simulink model "dinamica_quad"  (Simulink 7.6)
settings: Solver=ode45  StartTime=0.0  StopTime=10.0  MaxStep=0.1  RelTol=1e-3
values from neighbouring files (symbols this model uses):
  g = evalin('base','g')    [f.m]
  Ixx = evalin('base','Ixx')    [f.m]
  Iyy = evalin('base','Iyy')    [f.m]
  Izz = evalin('base','Izz')    [f.m]
  Izzm = evalin('base','Izzm')    [f.m]
  L = evalin('base','L')    [f.m]
  M = evalin('base','M')    [f.m]
  phi0 = evalin('base','phi0')    [determinar_vel.m]
  psi0 = evalin('base','psi0')    [determinar_vel.m]
  theta0 = evalin('base','theta0')    [determinar_vel.m]
undefined symbols (not defined in the file or in its folder): vq10, vq20, vq30, wq10, wq20, wq30, x0, y0, z0
settings Model: Creator=pater  LastModifiedBy=pater

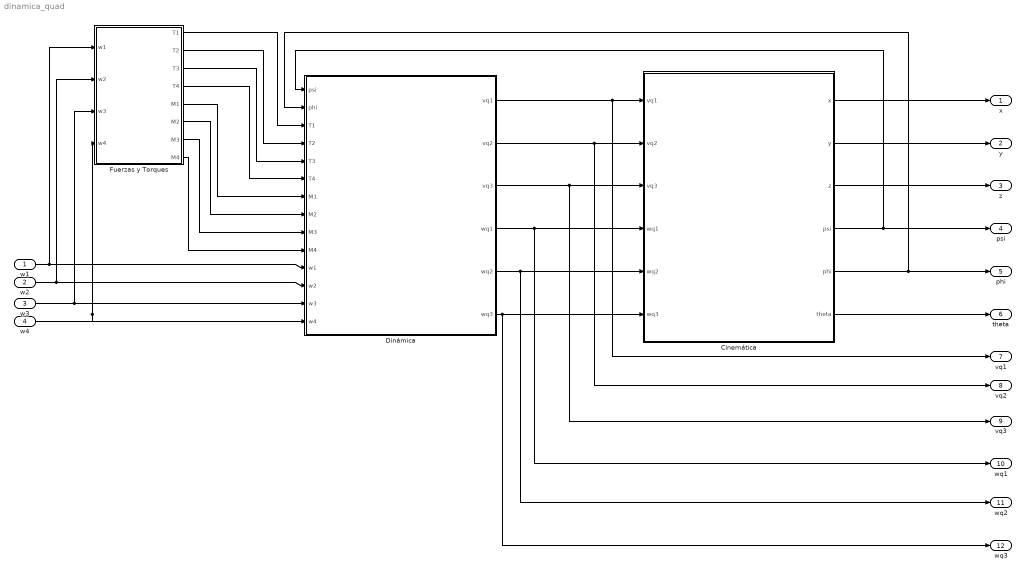
== system dinamica_quad ==
  w1 : Inport
  w2 : Inport  Port=2
  w3 : Inport  Port=3
  w4 : Inport  Port=4
  Cinemática : Subsystem
  Dinámica : Subsystem
  Fuerzas y Torques : Subsystem
  x : Outport
  y : Outport  Port=2
  z : Outport  Port=3
  psi : Outport  Port=4
  phi : Outport  Port=5
  theta : Outport  Port=6
  vq1 : Outport  Port=7
  vq2 : Outport  Port=8
  vq3 : Outport  Port=9
  wq1 : Outport  Port=10
  wq2 : Outport  Port=11
  wq3 : Outport  Port=12
  wires:
  Cinemática/1(x) -> x/1
  Cinemática/2(y) -> y/1
  Cinemática/3(z) -> z/1
  Cinemática/4(psi) -> psi/1, Dinámica/1(psi)
  Cinemática/5(phi) -> phi/1, Dinámica/2(phi)
  Cinemática/6(theta) -> theta/1
  w2/1 -> Fuerzas y Torques/2(w2), Dinámica/12(w2)
  w3/1 -> Fuerzas y Torques/3(w3), Dinámica/13(w3)
  w4/1 -> Fuerzas y Torques/4(w4), Dinámica/14(w4)
  Dinámica/6(wq3) -> wq3/1, Cinemática/6(wq3)
  Fuerzas y Torques/1(T1) -> Dinámica/3(T1)
  Fuerzas y Torques/2(T2) -> Dinámica/4(T2)
  Fuerzas y Torques/3(T3) -> Dinámica/5(T3)
  Fuerzas y Torques/4(T4) -> Dinámica/6(T4)
  Fuerzas y Torques/5(M1) -> Dinámica/7(M1)
  Fuerzas y Torques/6(M2) -> Dinámica/8(M2)
  Fuerzas y Torques/7(M3) -> Dinámica/9(M3)
  Fuerzas y Torques/8(M4) -> Dinámica/10(M4)
  w1/1 -> Fuerzas y Torques/1(w1), Dinámica/11(w1)
  Dinámica/1(vq1) -> Cinemática/1(vq1), vq1/1
  Dinámica/2(vq2) -> Cinemática/2(vq2), vq2/1
  Dinámica/3(vq3) -> Cinemática/3(vq3), vq3/1
  Dinámica/4(wq1) -> Cinemática/4(wq1), wq1/1
  Dinámica/5(wq2) -> Cinemática/5(wq2), wq2/1

== system dinamica_quad/Cinemática ==
  vq1 : Inport
  vq2 : Inport  Port=2
  vq3 : Inport  Port=3
  wq1 : Inport  Port=4
  wq2 : Inport  Port=5
  wq3 : Inport  Port=6
  Posiciones : Subsystem
  Ángulos De Euler : Subsystem
  x : Outport
  y : Outport  Port=2
  z : Outport  Port=3
  psi : Outport  Port=4
  phi : Outport  Port=5
  theta : Outport  Port=6
  wires:
  Posiciones/1(x) -> x/1
  Posiciones/2(y) -> y/1
  Posiciones/3(z) -> z/1
  Ángulos De Euler/1(psi) -> psi/1, Posiciones/3(psi)
  Ángulos De Euler/2(phi) -> phi/1, Posiciones/2(phi)
  Ángulos De Euler/3(theta) -> theta/1, Posiciones/1(theta)
  vq1/1 -> Posiciones/4(vq1)
  vq2/1 -> Posiciones/5(vq2)
  vq3/1 -> Posiciones/6(vq3)
  wq1/1 -> Ángulos De Euler/1(wq1)
  wq2/1 -> Ángulos De Euler/2(wq2)
  wq3/1 -> Ángulos De Euler/3(wq3)

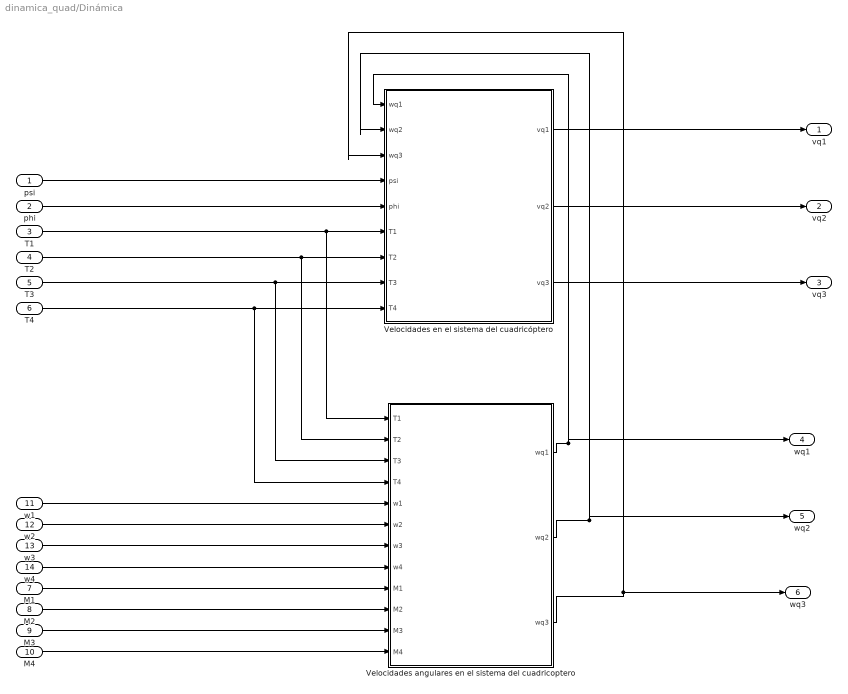
== system dinamica_quad/Dinámica ==
  psi : Inport
  phi : Inport  Port=2
  T1 : Inport  Port=3
  T2 : Inport  Port=4
  T3 : Inport  Port=5
  T4 : Inport  Port=6
  M1 : Inport  Port=7
  M2 : Inport  Port=8
  M3 : Inport  Port=9
  M4 : Inport  Port=10
  w1 : Inport  Port=11
  w2 : Inport  Port=12
  w3 : Inport  Port=13
  w4 : Inport  Port=14
  Velocidades angulares en el sistema del cuadricoptero : Subsystem
  Velocidades en el sistema del cuadricóptero : Subsystem
  vq1 : Outport
  vq2 : Outport  Port=2
  vq3 : Outport  Port=3
  wq1 : Outport  Port=4
  wq2 : Outport  Port=5
  wq3 : Outport  Port=6
  wires:
  T1/1 -> Velocidades en el sistema del cuadricóptero/6(T1), Velocidades angulares en el sistema del cuadricoptero/1(T1)
  T2/1 -> Velocidades en el sistema del cuadricóptero/7(T2), Velocidades angulares en el sistema del cuadricoptero/2(T2)
  T3/1 -> Velocidades en el sistema del cuadricóptero/8(T3), Velocidades angulares en el sistema del cuadricoptero/3(T3)
  T4/1 -> Velocidades en el sistema del cuadricóptero/9(T4), Velocidades angulares en el sistema del cuadricoptero/4(T4)
  Velocidades angulares en el sistema del cuadricoptero/1(wq1) -> wq1/1, Velocidades en el sistema del cuadricóptero/1(wq1)
  Velocidades angulares en el sistema del cuadricoptero/2(wq2) -> wq2/1, Velocidades en el sistema del cuadricóptero/2(wq2)
  Velocidades angulares en el sistema del cuadricoptero/3(wq3) -> Velocidades en el sistema del cuadricóptero/3(wq3), wq3/1
  phi/1 -> Velocidades en el sistema del cuadricóptero/5(phi)
  psi/1 -> Velocidades en el sistema del cuadricóptero/4(psi)
  Velocidades en el sistema del cuadricóptero/3(vq3) -> vq3/1
  Velocidades en el sistema del cuadricóptero/2(vq2) -> vq2/1
  Velocidades en el sistema del cuadricóptero/1(vq1) -> vq1/1
  M2/1 -> Velocidades angulares en el sistema del cuadricoptero/10(M2)
  M3/1 -> Velocidades angulares en el sistema del cuadricoptero/11(M3)
  M4/1 -> Velocidades angulares en el sistema del cuadricoptero/12(M4)
  M1/1 -> Velocidades angulares en el sistema del cuadricoptero/9(M1)
  w1/1 -> Velocidades angulares en el sistema del cuadricoptero/5(w1)
  w2/1 -> Velocidades angulares en el sistema del cuadricoptero/6(w2)
  w3/1 -> Velocidades angulares en el sistema del cuadricoptero/7(w3)
  w4/1 -> Velocidades angulares en el sistema del cuadricoptero/8(w4)

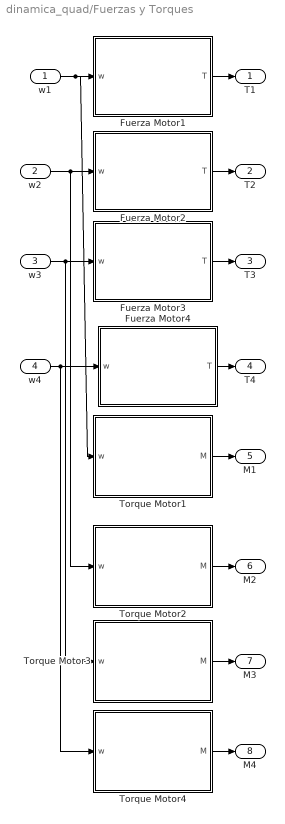
== system dinamica_quad/Fuerzas y Torques ==
  w1 : Inport
  w2 : Inport  Port=2
  w3 : Inport  Port=3
  w4 : Inport  Port=4
  Fuerza Motor1 : Subsystem
  Fuerza Motor2 : Subsystem
  Fuerza Motor3 : Subsystem
  Fuerza Motor4 : Subsystem
  Torque Motor1 : Subsystem
  Torque Motor2 : Subsystem
  Torque Motor3 : Subsystem
  Torque Motor4 : Subsystem
  T1 : Outport
  T2 : Outport  Port=2
  T3 : Outport  Port=3
  T4 : Outport  Port=4
  M1 : Outport  Port=5
  M2 : Outport  Port=6
  M3 : Outport  Port=7
  M4 : Outport  Port=8
  wires:
  w1/1 -> Fuerza Motor1/1(w), Torque Motor1/1(w)
  w2/1 -> Fuerza Motor2/1(w), Torque Motor2/1(w)
  w3/1 -> Fuerza Motor3/1(w), Torque Motor3/1(w)
  w4/1 -> Fuerza Motor4/1(w), Torque Motor4/1(w)
  Fuerza Motor1/1(T) -> T1/1
  Fuerza Motor2/1(T) -> T2/1
  Fuerza Motor3/1(T) -> T3/1
  Fuerza Motor4/1(T) -> T4/1
  Torque Motor1/1(M) -> M1/1
  Torque Motor2/1(M) -> M2/1
  Torque Motor3/1(M) -> M3/1
  Torque Motor4/1(M) -> M4/1

== system dinamica_quad/Cinemática/Posiciones ==
  theta : Inport
  phi : Inport  Port=2
  psi : Inport  Port=3
  vq1 : Inport  Port=4
  vq2 : Inport  Port=5
  vq3 : Inport  Port=6
  Subsystem3 : Subsystem
  Subsystem4 : Subsystem
  Subsystem5 : Subsystem
  x : Outport
  y : Outport  Port=2
  z : Outport  Port=3
  wires:
  Subsystem3/1(x) -> x/1
  Subsystem4/1(y) -> y/1
  Subsystem5/1(z) -> z/1
  vq3/1 -> Subsystem5/5(vq3), Subsystem4/6(vq3), Subsystem3/6(vq3)
  theta/1 -> Subsystem3/1(theta), Subsystem4/1(theta)
  phi/1 -> Subsystem3/2(phi), Subsystem4/2(phi), Subsystem5/1(phi)
  psi/1 -> Subsystem3/3(psi), Subsystem4/3(psi), Subsystem5/2(psi)
  vq2/1 -> Subsystem5/4(vq2), Subsystem4/5(vq2), Subsystem3/5(vq2)
  vq1/1 -> Subsystem5/3(vq1), Subsystem4/4(vq1), Subsystem3/4(vq1)

== system dinamica_quad/Cinemática/Ángulos De Euler ==
  wq1 : Inport
  wq2 : Inport  Port=2
  wq3 : Inport  Port=3
  Subsystem : Subsystem
  Subsystem1 : Subsystem
  Subsystem2 : Subsystem
  psi : Outport
  phi : Outport  Port=2
  theta : Outport  Port=3
  wires:
  Subsystem1/1(psi) -> psi/1, Subsystem/1(psi), Subsystem2/1(psi)
  Subsystem2/1(phi) -> phi/1, Subsystem/2(phi), Subsystem1/1(phi)
  Subsystem/1(theta) -> theta/1
  wq3/1 -> Subsystem/4(wq3), Subsystem2/3(wq3), Subsystem1/2(wq3)
  wq1/1 -> Subsystem1/4(wq1)
  wq2/1 -> Subsystem2/2(wq2), Subsystem1/3(wq2), Subsystem/3(wq2)

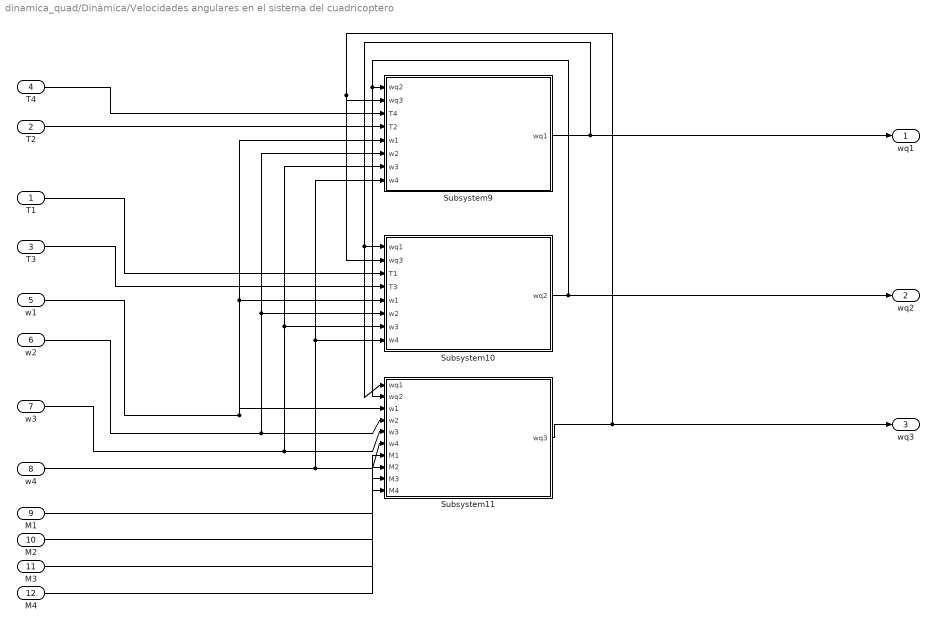
== system dinamica_quad/Dinámica/Velocidades angulares en el sistema del cuadricoptero ==
  T1 : Inport
  T2 : Inport  Port=2
  T3 : Inport  Port=3
  T4 : Inport  Port=4
  w1 : Inport  Port=5
  w2 : Inport  Port=6
  w3 : Inport  Port=7
  w4 : Inport  Port=8
  M1 : Inport  Port=9
  M2 : Inport  Port=10
  M3 : Inport  Port=11
  M4 : Inport  Port=12
  Subsystem10 : Subsystem
  Subsystem11 : Subsystem
  Subsystem9 : Subsystem
  wq1 : Outport
  wq2 : Outport  Port=2
  wq3 : Outport  Port=3
  wires:
  Subsystem9/1(wq1) -> wq1/1, Subsystem11/1(wq1), Subsystem10/1(wq1)
  Subsystem10/1(wq2) -> wq2/1, Subsystem11/2(wq2), Subsystem9/1(wq2)
  Subsystem11/1(wq3) -> wq3/1, Subsystem10/2(wq3), Subsystem9/2(wq3)
  w4/1 -> Subsystem11/6(w4), Subsystem10/8(w4), Subsystem9/8(w4)
  w3/1 -> Subsystem11/5(w3), Subsystem10/7(w3), Subsystem9/7(w3)
  w2/1 -> Subsystem11/4(w2), Subsystem10/6(w2), Subsystem9/6(w2)
  w1/1 -> Subsystem11/3(w1), Subsystem10/5(w1), Subsystem9/5(w1)
  T3/1 -> Subsystem10/4(T3)
  T1/1 -> Subsystem10/3(T1)
  T2/1 -> Subsystem9/4(T2)
  T4/1 -> Subsystem9/3(T4)
  M1/1 -> Subsystem11/7(M1)
  M2/1 -> Subsystem11/8(M2)
  M3/1 -> Subsystem11/9(M3)
  M4/1 -> Subsystem11/10(M4)

== system dinamica_quad/Dinámica/Velocidades en el sistema del cuadricóptero ==
  wq1 : Inport
  wq2 : Inport  Port=2
  wq3 : Inport  Port=3
  psi : Inport  Port=4
  phi : Inport  Port=5
  T1 : Inport  Port=6
  T2 : Inport  Port=7
  T3 : Inport  Port=8
  T4 : Inport  Port=9
  Subsystem6 : Subsystem
  Subsystem7 : Subsystem
  Subsystem8 : Subsystem
  vq1 : Outport
  vq2 : Outport  Port=2
  vq3 : Outport  Port=3
  wires:
  Subsystem6/1(vq1) -> vq1/1, Subsystem8/5(vq1), Subsystem7/7(vq1), Subsystem7/8(vq2)
  Subsystem8/1(vq2) -> Subsystem6/4(vq2), vq2/1
  Subsystem7/1(vq3) -> vq3/1, Subsystem6/5(vq3), Subsystem8/4(vq3)
  wq1/1 -> Subsystem8/3(wq1), Subsystem7/1(wq1)
  wq3/1 -> Subsystem6/3(wq3), Subsystem8/2(wq3)
  psi/1 -> Subsystem8/6(psi), Subsystem7/10(psi)
  phi/1 -> Subsystem6/1(phi), Subsystem8/1(phi), Subsystem7/9(phi)
  wq2/1 -> Subsystem6/2(wq2), Subsystem7/2(wq2)
  T1/1 -> Subsystem7/3(T1)
  T2/1 -> Subsystem7/4(T2)
  T3/1 -> Subsystem7/5(T3)
  T4/1 -> Subsystem7/6(T4)

== system dinamica_quad/Fuerzas y Torques/Fuerza Motor1 ==
  w : Inport
  Add : Sum
  Gain : Gain  Gain=3.5296e-5
  Gain1 : Gain  Gain=-4.9293e-4
  Product : Product  RndMeth=Zero
  T : Outport
  wires:
  Add/1 -> T/1
  Gain1/1 -> Add/2
  Product/1 -> Gain/1
  Gain/1 -> Add/1
  w/1 -> Gain1/1, Product/2, Product/1

== system dinamica_quad/Fuerzas y Torques/Fuerza Motor2 ==
  w : Inport
  Add : Sum
  Gain : Gain  Gain=3.5296e-5
  Gain1 : Gain  Gain=-4.9293e-4
  Product : Product  RndMeth=Zero
  T : Outport
  wires:
  Add/1 -> T/1
  Gain1/1 -> Add/2
  Product/1 -> Gain/1
  Gain/1 -> Add/1
  w/1 -> Gain1/1, Product/2, Product/1

== system dinamica_quad/Fuerzas y Torques/Fuerza Motor3 ==
  w : Inport
  Add : Sum
  Gain : Gain  Gain=3.5296e-5
  Gain1 : Gain  Gain=-4.9293e-4
  Product : Product  RndMeth=Zero
  T : Outport
  wires:
  Add/1 -> T/1
  Gain1/1 -> Add/2
  Product/1 -> Gain/1
  Gain/1 -> Add/1
  w/1 -> Gain1/1, Product/2, Product/1

== system dinamica_quad/Fuerzas y Torques/Fuerza Motor4 ==
  w : Inport
  Add : Sum
  Gain : Gain  Gain=3.5296e-5
  Gain1 : Gain  Gain=-4.9293e-4
  Product : Product  RndMeth=Zero
  T : Outport
  wires:
  Add/1 -> T/1
  Gain1/1 -> Add/2
  Product/1 -> Gain/1
  Gain/1 -> Add/1
  w/1 -> Gain1/1, Product/2, Product/1

== system dinamica_quad/Fuerzas y Torques/Torque Motor1 ==
  w : Inport
  Add : Sum
  Gain : Gain  Gain=3.4734e-6
  Gain1 : Gain  Gain=-1.3205e-4
  Product : Product  RndMeth=Zero
  M : Outport
  wires:
  Add/1 -> M/1
  Gain1/1 -> Add/2
  Product/1 -> Gain/1
  Gain/1 -> Add/1
  w/1 -> Gain1/1, Product/2, Product/1

== system dinamica_quad/Fuerzas y Torques/Torque Motor2 ==
  w : Inport
  Add : Sum
  Gain : Gain  Gain=3.4734e-6
  Gain1 : Gain  Gain=-1.3205e-4
  Product : Product  RndMeth=Zero
  M : Outport
  wires:
  Add/1 -> M/1
  Gain1/1 -> Add/2
  Product/1 -> Gain/1
  Gain/1 -> Add/1
  w/1 -> Gain1/1, Product/2, Product/1

== system dinamica_quad/Fuerzas y Torques/Torque Motor3 ==
  w : Inport
  Add : Sum
  Gain : Gain  Gain=3.4734e-6
  Gain1 : Gain  Gain=-1.3205e-4
  Product : Product  RndMeth=Zero
  M : Outport
  wires:
  Add/1 -> M/1
  Gain1/1 -> Add/2
  Product/1 -> Gain/1
  Gain/1 -> Add/1
  w/1 -> Gain1/1, Product/2, Product/1

== system dinamica_quad/Fuerzas y Torques/Torque Motor4 ==
  w : Inport
  Add : Sum
  Gain : Gain  Gain=3.4734e-6
  Gain1 : Gain  Gain=-1.3205e-4
  Product : Product  RndMeth=Zero
  M : Outport
  wires:
  Add/1 -> M/1
  Gain1/1 -> Add/2
  Product/1 -> Gain/1
  Gain/1 -> Add/1
  w/1 -> Gain1/1, Product/2, Product/1

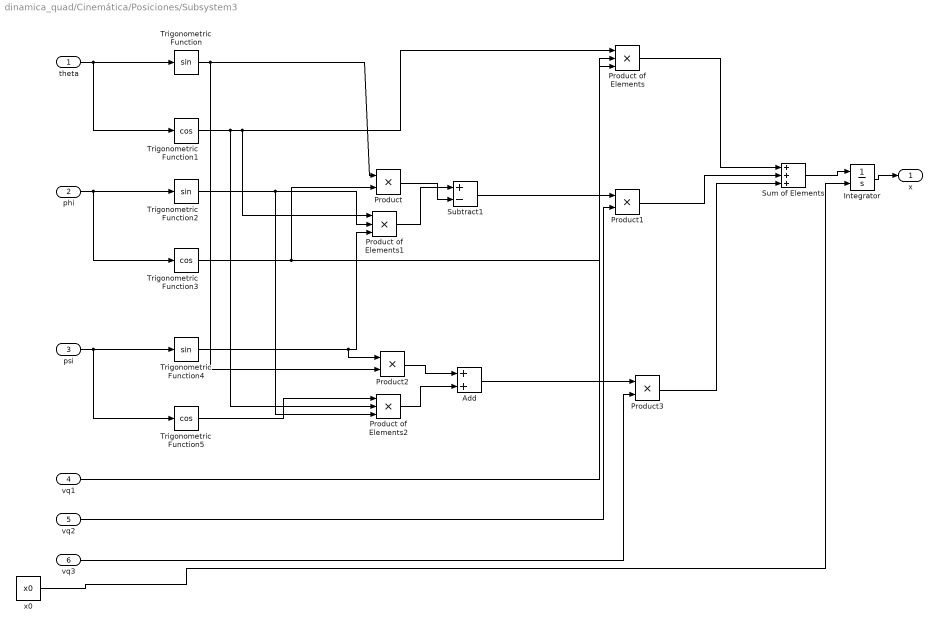
== system dinamica_quad/Cinemática/Posiciones/Subsystem3 ==
  theta : Inport
  phi : Inport  Port=2
  psi : Inport  Port=3
  vq1 : Inport  Port=4
  vq2 : Inport  Port=5
  vq3 : Inport  Port=6
  Add : Sum
  Integrator : Integrator  InitialConditionSource=external
  Product{,1..3} (4 alike) : Product  RndMeth=Zero
  Product of Elements : Product  Inputs=3
  Product of Elements1 : Product  Inputs=3
  Product of Elements2 : Product  Inputs=3
  Subtract1 : Sum  Inputs=+-
  Sum of Elements : Sum  Inputs=3
  Trigonometric Function : Trigonometry
  Trigonometric Function1 : Trigonometry  Operator=cos
  Trigonometric Function2 : Trigonometry
  Trigonometric Function3 : Trigonometry  Operator=cos
  Trigonometric Function4 : Trigonometry
  Trigonometric Function5 : Trigonometry  Operator=cos
  x0 : Constant  Value=x0
  x : Outport
  wires:
  theta/1 -> Trigonometric Function/1, Trigonometric Function1/1
  phi/1 -> Trigonometric Function2/1, Trigonometric Function3/1
  psi/1 -> Trigonometric Function4/1, Trigonometric Function5/1
  Trigonometric Function1/1 -> Product of Elements/1, Product of Elements1/1, Product of Elements2/2
  Trigonometric Function3/1 -> Product of Elements/2, Product/2
  vq1/1 -> Product of Elements/3
  Trigonometric Function/1 -> Product/1, Product2/2
  Trigonometric Function2/1 -> Product of Elements1/2, Product of Elements2/3
  Trigonometric Function4/1 -> Product of Elements1/3, Product2/1
  Subtract1/1 -> Product1/1
  vq2/1 -> Product1/2
  Product2/1 -> Add/1
  Product of Elements2/1 -> Add/2
  Trigonometric Function5/1 -> Product of Elements2/1
  Add/1 -> Product3/1
  vq3/1 -> Product3/2
  Product of Elements/1 -> Sum of Elements/1
  Product1/1 -> Sum of Elements/2
  Product3/1 -> Sum of Elements/3
  Sum of Elements/1 -> Integrator/1
  Integrator/1 -> x/1
  Product of Elements1/1 -> Subtract1/1
  Product/1 -> Subtract1/2
  x0/1 -> Integrator/2

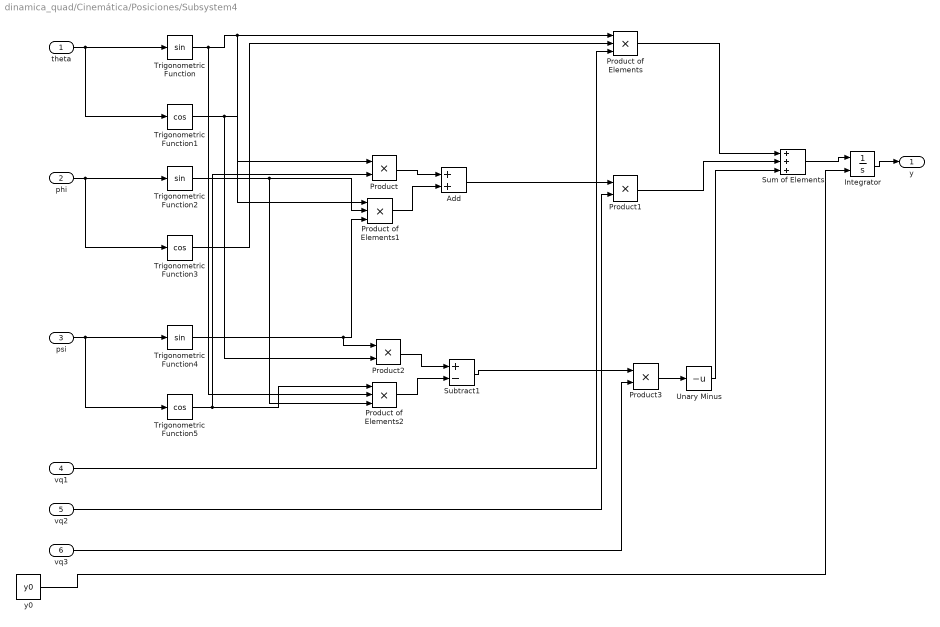
== system dinamica_quad/Cinemática/Posiciones/Subsystem4 ==
  theta : Inport
  phi : Inport  Port=2
  psi : Inport  Port=3
  vq1 : Inport  Port=4
  vq2 : Inport  Port=5
  vq3 : Inport  Port=6
  Add : Sum
  Integrator : Integrator  InitialConditionSource=external
  Product{,1..3} (4 alike) : Product  RndMeth=Zero
  Product of Elements : Product  Inputs=3
  Product of Elements1 : Product  Inputs=3
  Product of Elements2 : Product  Inputs=3
  Subtract1 : Sum  Inputs=+-
  Sum of Elements : Sum  Inputs=3
  Trigonometric Function : Trigonometry
  Trigonometric Function1 : Trigonometry  Operator=cos
  Trigonometric Function2 : Trigonometry
  Trigonometric Function3 : Trigonometry  Operator=cos
  Trigonometric Function4 : Trigonometry
  Trigonometric Function5 : Trigonometry  Operator=cos
  Unary Minus : UnaryMinus
  y0 : Constant  Value=y0
  y : Outport
  wires:
  theta/1 -> Trigonometric Function/1, Trigonometric Function1/1
  phi/1 -> Trigonometric Function2/1, Trigonometric Function3/1
  psi/1 -> Trigonometric Function4/1, Trigonometric Function5/1
  Trigonometric Function1/1 -> Product/1, Product2/2
  Trigonometric Function3/1 -> Product of Elements/2
  vq1/1 -> Product of Elements/3
  Trigonometric Function/1 -> Product of Elements/1, Product of Elements1/1, Product of Elements2/2
  Trigonometric Function2/1 -> Product of Elements1/2, Product of Elements2/3
  Trigonometric Function4/1 -> Product of Elements1/3, Product2/1
  Product/1 -> Add/1
  Product of Elements1/1 -> Add/2
  Add/1 -> Product1/1
  vq2/1 -> Product1/2
  Trigonometric Function5/1 -> Product of Elements2/1, Product/2
  Subtract1/1 -> Product3/1
  vq3/1 -> Product3/2
  Product of Elements/1 -> Sum of Elements/1
  Product1/1 -> Sum of Elements/2
  Product3/1 -> Unary Minus/1
  Sum of Elements/1 -> Integrator/1
  Integrator/1 -> y/1
  Unary Minus/1 -> Sum of Elements/3
  Product of Elements2/1 -> Subtract1/2
  Product2/1 -> Subtract1/1
  y0/1 -> Integrator/2

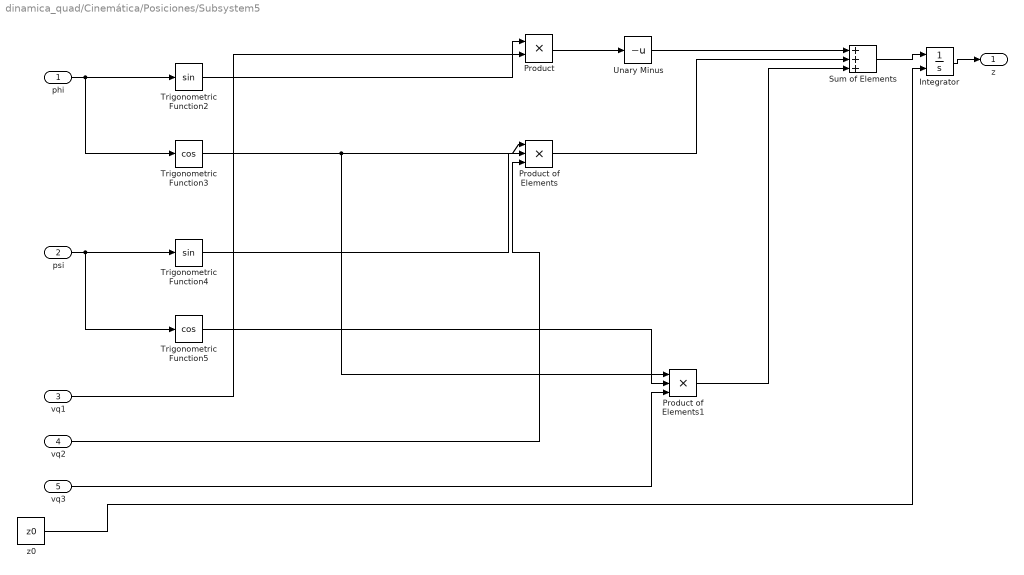
== system dinamica_quad/Cinemática/Posiciones/Subsystem5 ==
  phi : Inport
  psi : Inport  Port=2
  vq1 : Inport  Port=3
  vq2 : Inport  Port=4
  vq3 : Inport  Port=5
  Integrator : Integrator  InitialConditionSource=external
  Product : Product  RndMeth=Zero
  Product of Elements : Product  Inputs=3
  Product of Elements1 : Product  Inputs=3
  Sum of Elements : Sum  Inputs=3
  Trigonometric Function2 : Trigonometry
  Trigonometric Function3 : Trigonometry  Operator=cos
  Trigonometric Function4 : Trigonometry
  Trigonometric Function5 : Trigonometry  Operator=cos
  Unary Minus : UnaryMinus
  z0 : Constant  Value=z0
  z : Outport
  wires:
  phi/1 -> Trigonometric Function2/1, Trigonometric Function3/1
  psi/1 -> Trigonometric Function4/1, Trigonometric Function5/1
  Sum of Elements/1 -> Integrator/1
  Integrator/1 -> z/1
  Trigonometric Function2/1 -> Product/1
  vq1/1 -> Product/2
  Product/1 -> Unary Minus/1
  Trigonometric Function3/1 -> Product of Elements/1, Product of Elements1/1
  Trigonometric Function4/1 -> Product of Elements/2
  vq2/1 -> Product of Elements/3
  Trigonometric Function5/1 -> Product of Elements1/2
  vq3/1 -> Product of Elements1/3
  Product of Elements/1 -> Sum of Elements/2
  Product of Elements1/1 -> Sum of Elements/3
  Unary Minus/1 -> Sum of Elements/1
  z0/1 -> Integrator/2

== system dinamica_quad/Cinemática/Ángulos De Euler/Subsystem ==
  psi : Inport
  phi : Inport  Port=2
  wq2 : Inport  Port=3
  wq3 : Inport  Port=4
  Divide : Product  Inputs=*/
  Integrator : Integrator  InitialConditionSource=external
  Product : Product  RndMeth=Zero
  Product1 : Product  RndMeth=Zero
  Sum : Sum  Inputs=|++
  Trigonometric Function : Trigonometry  Operator=cos
  Trigonometric Function1 : Trigonometry
  Trigonometric Function2 : Trigonometry  Operator=cos
  theta0 : Constant  Value=theta0
  theta : Outport
  wires:
  wq3/1 -> Product/1
  wq2/1 -> Product1/1
  Product/1 -> Sum/1
  Product1/1 -> Sum/2
  Sum/1 -> Divide/1
  Trigonometric Function2/1 -> Divide/2
  Divide/1 -> Integrator/1
  Trigonometric Function/1 -> Product/2
  Trigonometric Function1/1 -> Product1/2
  phi/1 -> Trigonometric Function2/1
  Integrator/1 -> theta/1
  psi/1 -> Trigonometric Function/1, Trigonometric Function1/1
  theta0/1 -> Integrator/2

== system dinamica_quad/Cinemática/Ángulos De Euler/Subsystem1 ==
  phi : Inport
  wq3 : Inport  Port=2
  wq2 : Inport  Port=3
  wq1 : Inport  Port=4
  Add : Sum
  Integrator : Integrator  InitialConditionSource=external
  Product : Product  RndMeth=Zero
  Product1 : Product  RndMeth=Zero
  Product2 : Product  RndMeth=Zero
  Sum : Sum  Inputs=|++
  Trigonometric Function : Trigonometry
  Trigonometric Function2 : Trigonometry  Operator=tan
  Trigonometric Function3 : Trigonometry  Operator=cos
  psi0 : Constant  Value=psi0
  psi : Outport
  wires:
  Integrator/1 -> psi/1, Trigonometric Function3/1, Trigonometric Function/1
  Product/1 -> Sum/1
  phi/1 -> Trigonometric Function2/1
  Trigonometric Function2/1 -> Product/2
  wq3/1 -> Product1/2
  Trigonometric Function3/1 -> Product1/1
  Product1/1 -> Add/1
  Add/1 -> Product/1
  Trigonometric Function/1 -> Product2/1
  wq2/1 -> Product2/2
  Product2/1 -> Add/2
  wq1/1 -> Sum/2
  Sum/1 -> Integrator/1
  psi0/1 -> Integrator/2

== system dinamica_quad/Cinemática/Ángulos De Euler/Subsystem2 ==
  psi : Inport
  wq2 : Inport  Port=2
  wq3 : Inport  Port=3
  Integrator : Integrator  InitialConditionSource=external
  Product : Product  RndMeth=Zero
  Product1 : Product  RndMeth=Zero
  Subtract : Sum  Inputs=+-
  Trigonometric Function : Trigonometry  Operator=cos
  Trigonometric Function1 : Trigonometry
  phi0 : Constant  Value=phi0
  phi : Outport
  wires:
  Integrator/1 -> phi/1
  Subtract/1 -> Integrator/1
  Product/1 -> Subtract/1
  Product1/1 -> Subtract/2
  Trigonometric Function/1 -> Product/1
  psi/1 -> Trigonometric Function/1, Trigonometric Function1/1
  Trigonometric Function1/1 -> Product1/1
  wq2/1 -> Product/2
  wq3/1 -> Product1/2
  phi0/1 -> Integrator/2

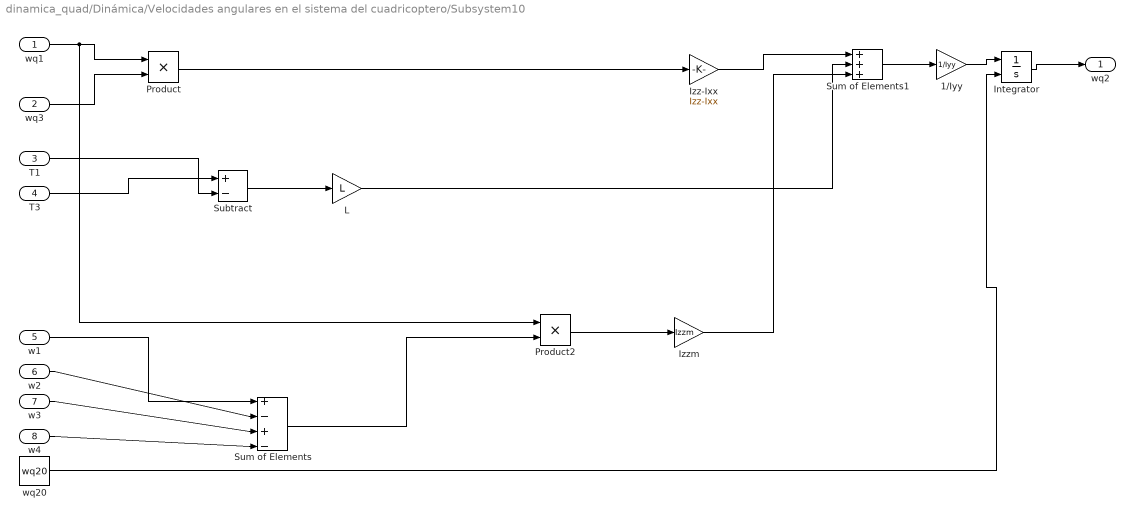
== system dinamica_quad/Dinámica/Velocidades angulares en el sistema del cuadricoptero/Subsystem10 ==
  wq1 : Inport
  wq3 : Inport  Port=2
  T1 : Inport  Port=3
  T3 : Inport  Port=4
  w1 : Inport  Port=5
  w2 : Inport  Port=6
  w3 : Inport  Port=7
  w4 : Inport  Port=8
  1/Iyy : Gain  Gain=1/Iyy
  Integrator : Integrator  InitialConditionSource=external
  Izz-Ixx : Gain  Gain=Izz-Ixx
  Izzm : Gain  Gain=Izzm
  L : Gain  Gain=L
  Product : Product  RndMeth=Zero
  Product2 : Product  RndMeth=Zero
  Subtract : Sum  Inputs=+-
  Sum of Elements : Sum  Inputs=+|-|+|-|
  Sum of Elements1 : Sum  Inputs=3
  wq20 : Constant  Value=wq20
  wq2 : Outport
  wires:
  wq1/1 -> Product/1, Product2/1
  wq3/1 -> Product/2
  Product/1 -> Izz-Ixx/1
  T3/1 -> Subtract/1
  T1/1 -> Subtract/2
  w1/1 -> Sum of Elements/1
  w2/1 -> Sum of Elements/2
  w3/1 -> Sum of Elements/3
  w4/1 -> Sum of Elements/4
  Sum of Elements/1 -> Product2/2
  Product2/1 -> Izzm/1
  Izzm/1 -> Sum of Elements1/3
  Sum of Elements1/1 -> 1/Iyy/1
  1/Iyy/1 -> Integrator/1
  Integrator/1 -> wq2/1
  Subtract/1 -> L/1
  Izz-Ixx/1 -> Sum of Elements1/1
  L/1 -> Sum of Elements1/2
  wq20/1 -> Integrator/2

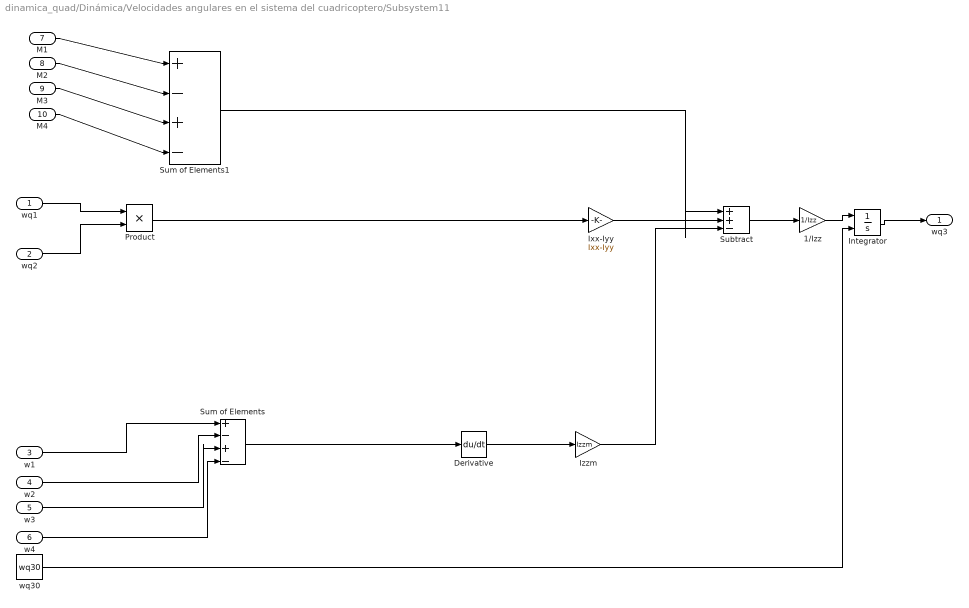
== system dinamica_quad/Dinámica/Velocidades angulares en el sistema del cuadricoptero/Subsystem11 ==
  wq1 : Inport
  wq2 : Inport  Port=2
  w1 : Inport  Port=3
  w2 : Inport  Port=4
  w3 : Inport  Port=5
  w4 : Inport  Port=6
  M1 : Inport  Port=7
  M2 : Inport  Port=8
  M3 : Inport  Port=9
  M4 : Inport  Port=10
  1/Izz : Gain  Gain=1/Izz
  Derivative : Derivative
  Integrator : Integrator  InitialConditionSource=external
  Ixx-Iyy : Gain  Gain=Ixx-Iyy
  Izzm : Gain  Gain=Izzm
  Product : Product  RndMeth=Zero
  Subtract : Sum  Inputs=++-
  Sum of Elements : Sum  Inputs=+|-|+|-|
  Sum of Elements1 : Sum  Inputs=+|-|+|-|
  wq30 : Constant  Value=wq30
  wq3 : Outport
  wires:
  wq1/1 -> Product/1
  wq2/1 -> Product/2
  Product/1 -> Ixx-Iyy/1
  w4/1 -> Sum of Elements/4
  Derivative/1 -> Izzm/1
  Subtract/1 -> 1/Izz/1
  1/Izz/1 -> Integrator/1
  Integrator/1 -> wq3/1
  wq30/1 -> Integrator/2
  w1/1 -> Sum of Elements/1
  w2/1 -> Sum of Elements/2
  w3/1 -> Sum of Elements/3
  Sum of Elements/1 -> Derivative/1
  M1/1 -> Sum of Elements1/1
  M2/1 -> Sum of Elements1/2
  M3/1 -> Sum of Elements1/3
  M4/1 -> Sum of Elements1/4
  Sum of Elements1/1 -> Subtract/1
  Izzm/1 -> Subtract/3
  Ixx-Iyy/1 -> Subtract/2

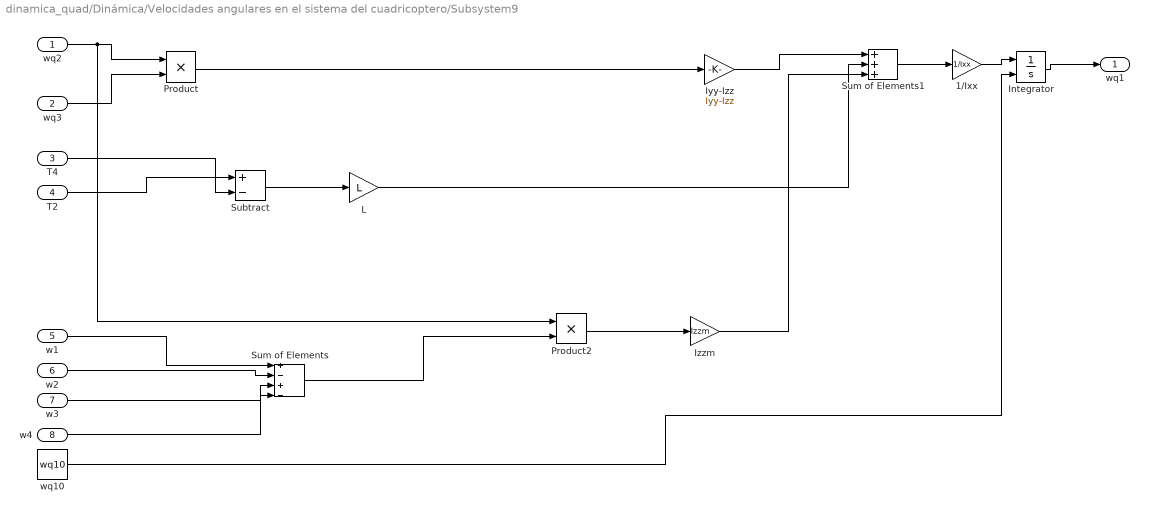
== system dinamica_quad/Dinámica/Velocidades angulares en el sistema del cuadricoptero/Subsystem9 ==
  wq2 : Inport
  wq3 : Inport  Port=2
  T4 : Inport  Port=3
  T2 : Inport  Port=4
  w1 : Inport  Port=5
  w2 : Inport  Port=6
  w3 : Inport  Port=7
  w4 : Inport  Port=8
  1/Ixx : Gain  Gain=1/Ixx
  Integrator : Integrator  InitialConditionSource=external
  Iyy-Izz : Gain  Gain=Iyy-Izz
  Izzm : Gain  Gain=Izzm
  L : Gain  Gain=L
  Product : Product  RndMeth=Zero
  Product2 : Product  RndMeth=Zero
  Subtract : Sum  Inputs=+-
  Sum of Elements : Sum  Inputs=+|-|+|-
  Sum of Elements1 : Sum  Inputs=3
  wq10 : Constant  Value=wq10
  wq1 : Outport
  wires:
  wq2/1 -> Product/1, Product2/1
  wq3/1 -> Product/2
  Product/1 -> Iyy-Izz/1
  T2/1 -> Subtract/1
  T4/1 -> Subtract/2
  w1/1 -> Sum of Elements/1
  w3/1 -> Sum of Elements/3
  w4/1 -> Sum of Elements/4
  Sum of Elements/1 -> Product2/2
  Product2/1 -> Izzm/1
  Izzm/1 -> Sum of Elements1/3
  Sum of Elements1/1 -> 1/Ixx/1
  1/Ixx/1 -> Integrator/1
  Integrator/1 -> wq1/1
  Subtract/1 -> L/1
  Iyy-Izz/1 -> Sum of Elements1/1
  L/1 -> Sum of Elements1/2
  w2/1 -> Sum of Elements/2
  wq10/1 -> Integrator/2

== system dinamica_quad/Dinámica/Velocidades en el sistema del cuadricóptero/Subsystem6 ==
  phi : Inport
  wq2 : Inport  Port=2
  wq3 : Inport  Port=3
  vq2 : Inport  Port=4
  vq3 : Inport  Port=5
  Add : Sum
  Integrator : Integrator  InitialConditionSource=external
  Product : Product  RndMeth=Zero
  Product1 : Product  RndMeth=Zero
  Subtract : Sum  Inputs=+-
  Trigonometric Function4 : Trigonometry
  gravedad : Gain  Gain=g
  vq10 : Constant  Value=vq10
  vq1 : Outport
  wires:
  phi/1 -> Trigonometric Function4/1
  vq2/1 -> Product/2
  wq3/1 -> Product/1
  vq3/1 -> Product1/2
  wq2/1 -> Product1/1
  Product/1 -> Subtract/1
  Product1/1 -> Subtract/2
  Trigonometric Function4/1 -> gravedad/1
  gravedad/1 -> Add/1
  Subtract/1 -> Add/2
  Add/1 -> Integrator/1
  Integrator/1 -> vq1/1
  vq10/1 -> Integrator/2

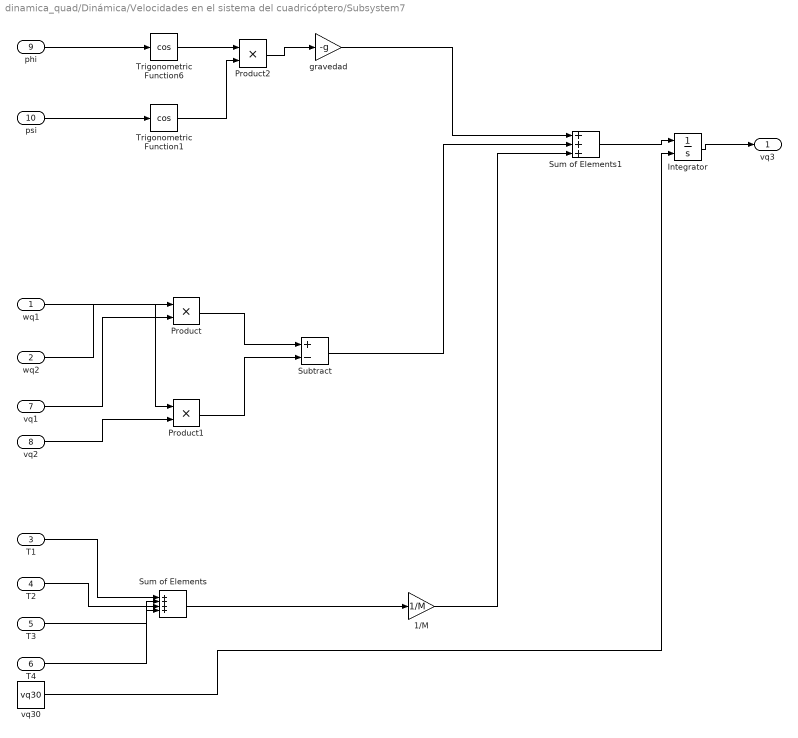
== system dinamica_quad/Dinámica/Velocidades en el sistema del cuadricóptero/Subsystem7 ==
  wq1 : Inport
  wq2 : Inport  Port=2
  T1 : Inport  Port=3
  T2 : Inport  Port=4
  T3 : Inport  Port=5
  T4 : Inport  Port=6
  vq1 : Inport  Port=7
  vq2 : Inport  Port=8
  phi : Inport  Port=9
  psi : Inport  Port=10
  1/M : Gain  Gain=1/M
  Integrator : Integrator  InitialConditionSource=external
  Product : Product  RndMeth=Zero
  Product1 : Product  RndMeth=Zero
  Product2 : Product  RndMeth=Zero
  Subtract : Sum  Inputs=+-
  Sum of Elements : Sum  Inputs=4
  Sum of Elements1 : Sum  Inputs=3
  Trigonometric Function1 : Trigonometry  Operator=cos
  Trigonometric Function6 : Trigonometry  Operator=cos
  gravedad : Gain  Gain=-g
  vq30 : Constant  Value=vq30
  vq3 : Outport
  wires:
  T1/1 -> Sum of Elements/1
  T2/1 -> Sum of Elements/2
  T3/1 -> Sum of Elements/3
  T4/1 -> Sum of Elements/4
  Sum of Elements/1 -> 1/M/1
  vq1/1 -> Product/2
  wq2/1 -> Product/1
  vq2/1 -> Product1/2
  wq1/1 -> Product1/1
  Product/1 -> Subtract/1
  Product1/1 -> Subtract/2
  phi/1 -> Trigonometric Function6/1
  psi/1 -> Trigonometric Function1/1
  Trigonometric Function1/1 -> Product2/2
  gravedad/1 -> Sum of Elements1/1
  Subtract/1 -> Sum of Elements1/2
  1/M/1 -> Sum of Elements1/3
  Sum of Elements1/1 -> Integrator/1
  Integrator/1 -> vq3/1
  Trigonometric Function6/1 -> Product2/1
  Product2/1 -> gravedad/1
  vq30/1 -> Integrator/2

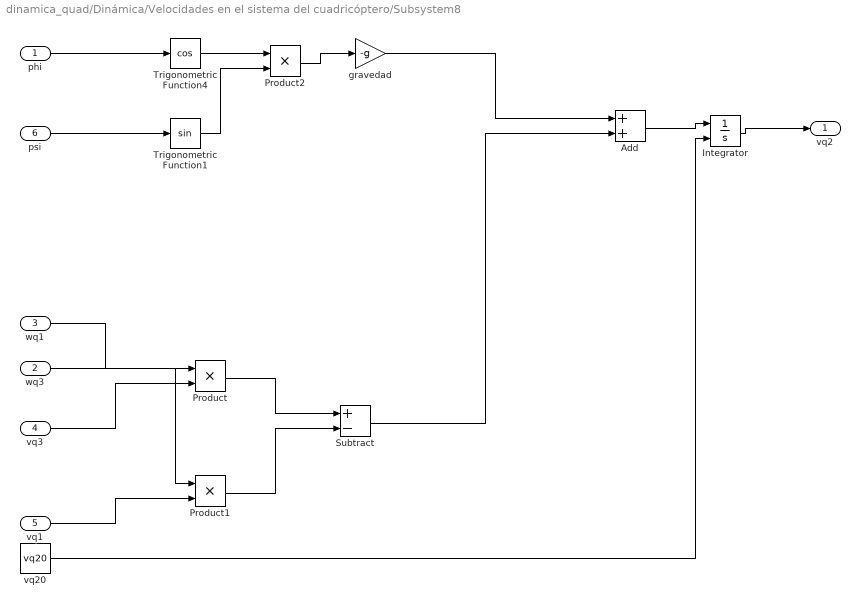
== system dinamica_quad/Dinámica/Velocidades en el sistema del cuadricóptero/Subsystem8 ==
  phi : Inport
  wq3 : Inport  Port=2
  wq1 : Inport  Port=3
  vq3 : Inport  Port=4
  vq1 : Inport  Port=5
  psi : Inport  Port=6
  Add : Sum
  Integrator : Integrator  InitialConditionSource=external
  Product : Product  RndMeth=Zero
  Product1 : Product  RndMeth=Zero
  Product2 : Product  RndMeth=Zero
  Subtract : Sum  Inputs=+-
  Trigonometric Function1 : Trigonometry
  Trigonometric Function4 : Trigonometry  Operator=cos
  gravedad : Gain  Gain=-g
  vq20 : Constant  Value=vq20
  vq2 : Outport
  wires:
  phi/1 -> Trigonometric Function4/1
  vq3/1 -> Product/2
  wq1/1 -> Product/1
  vq1/1 -> Product1/2
  wq3/1 -> Product1/1
  Product/1 -> Subtract/1
  Product1/1 -> Subtract/2
  gravedad/1 -> Add/1
  Subtract/1 -> Add/2
  Add/1 -> Integrator/1
  Integrator/1 -> vq2/1
  psi/1 -> Trigonometric Function1/1
  Trigonometric Function1/1 -> Product2/2
  Trigonometric Function4/1 -> Product2/1
  Product2/1 -> gravedad/1
  vq20/1 -> Integrator/2
